simulink library "INP_SPR_ManOver"  (R2024b)
settings: Solver=VariableStepAuto  StartTime=0.0  StopTime=10.0  RelTol=1e-3
undefined symbols (not defined in the file): INP_SPR_p_SwtAccSprFrLeMan_na, INP_SPR_p_SwtAccSprFrRiMan_na, INP_SPR_p_SwtAccSprReLeMan_na, INP_SPR_p_SwtAccSprReRiMan_na, INP_SPR_s_AccSprFrLeMan_mps2, INP_SPR_s_AccSprFrRiMan_mps2, INP_SPR_s_AccSprLoLimFrLe_mps2, INP_SPR_s_AccSprLoLimFrRi_mps2, INP_SPR_s_AccSprLoLimReLe_mps2, INP_SPR_s_AccSprLoLimReRi_mps2, INP_SPR_s_AccSprReLeMan_mps2, INP_SPR_s_AccSprReRiMan_mps2, INP_SPR_s_AccSprUpLimFrLe_mps2, INP_SPR_s_AccSprUpLimFrRi_mps2, INP_SPR_s_AccSprUpLimReLe_mps2, INP_SPR_s_AccSprUpLimReRi_mps2
libraries: simulink x4
settings Model: Creator=blatak  LastModifiedBy=jmbsp

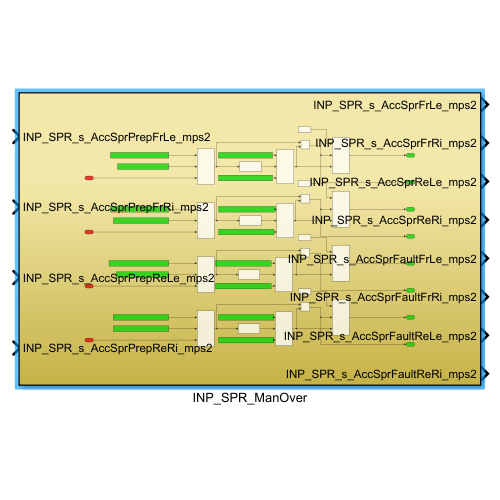
[thumbnail: Simulink's stored preview of the top-level diagram]
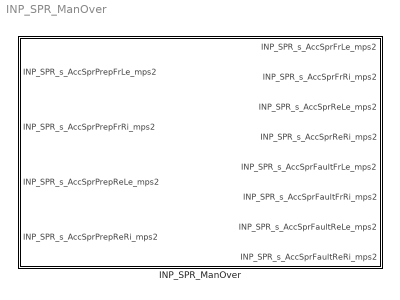
== system INP_SPR_ManOver ==
  INP_SPR_ManOver : Subsystem

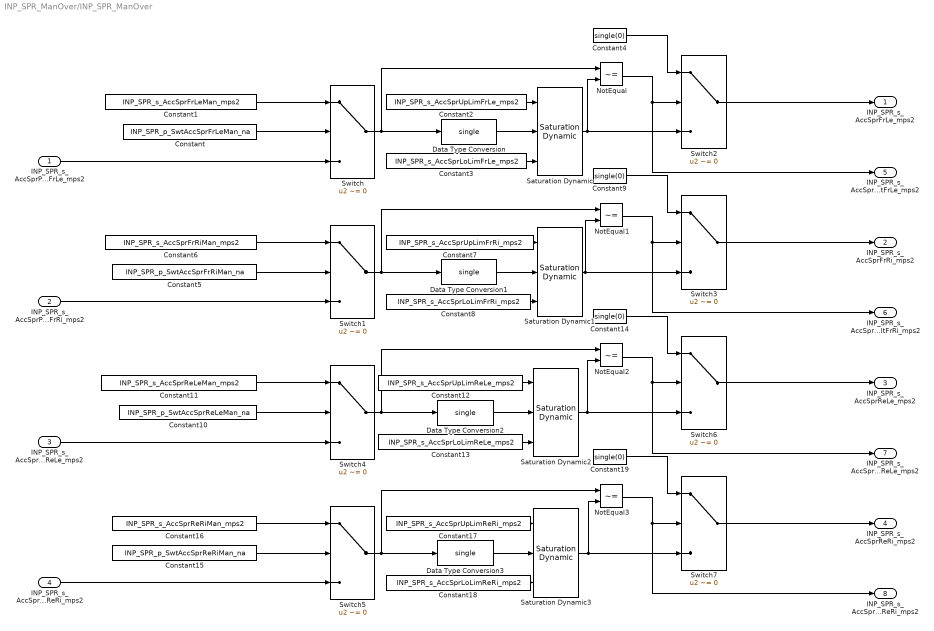
== system INP_SPR_ManOver/INP_SPR_ManOver ==
  INP_SPR_s_AccSprPrepFrLe_mps2 : Inport
  INP_SPR_s_AccSprPrepFrRi_mps2 : Inport  Port=2
  INP_SPR_s_AccSprPrepReLe_mps2 : Inport  Port=3
  INP_SPR_s_AccSprPrepReRi_mps2 : Inport  Port=4
  Constant : Constant  Description=|  Value=INP_SPR_p_SwtAccSprFrLeMan_na
      | Switch for manual override of the longitudinal acceleration value, if 1 instead the measured 
      | value the INP_IMU_p_ALgtVehMan_mps2 is used
  Constant1 : Constant  Description=|  Value=INP_SPR_s_AccSprFrLeMan_mps2
      | Value for longitudinal acceleration, which is used if the INP_IMU_p_SwtAXxxVehMan_na
      | is set to 1 instead of the measured value
  Constant10 : Constant  Description=|  Value=INP_SPR_p_SwtAccSprReLeMan_na
      | Switch for manual override of the longitudinal acceleration value, if 1 instead the measured 
      | value the INP_IMU_p_ALgtVehMan_mps2 is used
  Constant11 : Constant  Description=|  Value=INP_SPR_s_AccSprReLeMan_mps2
      | Value for longitudinal acceleration, which is used if the INP_IMU_p_SwtAXxxVehMan_na
      | is set to 1 instead of the measured value
  Constant12 : Constant  Description=Upper saturation limit for longitudinal acceleration  Value=INP_SPR_s_AccSprUpLimReLe_mps2
  Constant13 : Constant  Description=Lower saturation limit for longitudinal acceleration  Value=INP_SPR_s_AccSprLoLimReLe_mps2
  Constant{4,9,14,19} (4 alike) : Constant  Value=single(0)
  Constant15 : Constant  Description=|  Value=INP_SPR_p_SwtAccSprReRiMan_na
      | Switch for manual override of the longitudinal acceleration value, if 1 instead the measured 
      | value the INP_IMU_p_ALgtVehMan_mps2 is used
  Constant16 : Constant  Description=|  Value=INP_SPR_s_AccSprReRiMan_mps2
      | Value for longitudinal acceleration, which is used if the INP_IMU_p_SwtAXxxVehMan_na
      | is set to 1 instead of the measured value
  Constant17 : Constant  Description=Upper saturation limit for longitudinal acceleration  Value=INP_SPR_s_AccSprUpLimReRi_mps2
  Constant18 : Constant  Description=Lower saturation limit for longitudinal acceleration  Value=INP_SPR_s_AccSprLoLimReRi_mps2
  Constant2 : Constant  Description=Upper saturation limit for longitudinal acceleration  Value=INP_SPR_s_AccSprUpLimFrLe_mps2
  Constant3 : Constant  Description=Lower saturation limit for longitudinal acceleration  Value=INP_SPR_s_AccSprLoLimFrLe_mps2
  Constant5 : Constant  Description=|  Value=INP_SPR_p_SwtAccSprFrRiMan_na
      | Switch for manual override of the longitudinal acceleration value, if 1 instead the measured 
      | value the INP_IMU_p_ALgtVehMan_mps2 is used
  Constant6 : Constant  Description=|  Value=INP_SPR_s_AccSprFrRiMan_mps2
      | Value for longitudinal acceleration, which is used if the INP_IMU_p_SwtAXxxVehMan_na
      | is set to 1 instead of the measured value
  Constant7 : Constant  Description=Upper saturation limit for longitudinal acceleration  Value=INP_SPR_s_AccSprUpLimFrRi_mps2
  Constant8 : Constant  Description=Lower saturation limit for longitudinal acceleration  Value=INP_SPR_s_AccSprLoLimFrRi_mps2
  Data Type Conversion{,1..3} (4 alike) : DataTypeConversion  OutDataTypeStr=single  SaturateOnIntegerOverflow=off  RndMeth=Floor
  NotEqual{,1..3} (4 alike) : RelationalOperator  Operator=~=  OutDataTypeStr=boolean  RndMeth=Simplest  InputSameDT=off
  Saturation Dynamic{,1..3} (4 alike) : simulink/Discontinuities/Saturation Dynamic  OutMin=[]  OutMax=[]  OutDataTypeStr=Inherit: Same as second input  OutDataType=fixdt(1, 16)  OutScaling=2^-10  DoSatur=off
  Switch{,1..7} (8 alike) : Switch  Criteria=u2 ~= 0  SaturateOnIntegerOverflow=off  InputSameDT=off
  INP_SPR_s_AccSprFrLe_mps2 : Outport
  INP_SPR_s_AccSprFrRi_mps2 : Outport  Port=2
  INP_SPR_s_AccSprReLe_mps2 : Outport  Port=3
  INP_SPR_s_AccSprReRi_mps2 : Outport  Port=4
  INP_SPR_s_AccSprFaultFrLe_mps2 : Outport  Port=5
  INP_SPR_s_AccSprFaultFrRi_mps2 : Outport  Port=6
  INP_SPR_s_AccSprFaultReLe_mps2 : Outport  Port=7
  INP_SPR_s_AccSprFaultReRi_mps2 : Outport  Port=8
  wires:
  Constant7/1 -> Saturation Dynamic1/1
  NotEqual1/1 -> INP_SPR_s_AccSprFaultFrRi_mps2/1, Switch3/2
  Saturation Dynamic2/1 -> Switch6/3, NotEqual2/2
  Constant6/1 -> Switch1/1
  Data Type Conversion/1 -> Saturation Dynamic/2
  NotEqual/1 -> INP_SPR_s_AccSprFaultFrLe_mps2/1, Switch2/2
  INP_SPR_s_AccSprPrepReRi_mps2/1 -> Switch5/3
  Saturation Dynamic1/1 -> Switch3/3, NotEqual1/2
  Constant1/1 -> Switch/1
  NotEqual2/1 -> INP_SPR_s_AccSprFaultReLe_mps2/1, Switch6/2
  Constant13/1 -> Saturation Dynamic2/3
  Constant16/1 -> Switch5/1
  INP_SPR_s_AccSprPrepFrRi_mps2/1 -> Switch1/3
  Constant17/1 -> Saturation Dynamic3/1
  Switch4/1 -> NotEqual2/1, Data Type Conversion2/1
  Data Type Conversion2/1 -> Saturation Dynamic2/2
  Saturation Dynamic3/1 -> Switch7/3, NotEqual3/2
  Constant14/1 -> Switch6/1
  Constant10/1 -> Switch4/2
  Switch2/1 -> INP_SPR_s_AccSprFrLe_mps2/1
  Constant3/1 -> Saturation Dynamic/3
  Constant12/1 -> Saturation Dynamic2/1
  INP_SPR_s_AccSprPrepReLe_mps2/1 -> Switch4/3
  Saturation Dynamic/1 -> Switch2/3, NotEqual/2
  Switch6/1 -> INP_SPR_s_AccSprReLe_mps2/1
  Constant8/1 -> Saturation Dynamic1/3
  Switch1/1 -> NotEqual1/1, Data Type Conversion1/1
  Switch/1 -> NotEqual/1, Data Type Conversion/1
  Constant/1 -> Switch/2
  NotEqual3/1 -> INP_SPR_s_AccSprFaultReRi_mps2/1, Switch7/2
  Constant18/1 -> Saturation Dynamic3/3
  Constant2/1 -> Saturation Dynamic/1
  Switch5/1 -> NotEqual3/1, Data Type Conversion3/1
  Constant11/1 -> Switch4/1
  Data Type Conversion1/1 -> Saturation Dynamic1/2
  Data Type Conversion3/1 -> Saturation Dynamic3/2
  INP_SPR_s_AccSprPrepFrLe_mps2/1 -> Switch/3
  Constant15/1 -> Switch5/2
  Switch7/1 -> INP_SPR_s_AccSprReRi_mps2/1
  Switch3/1 -> INP_SPR_s_AccSprFrRi_mps2/1
  Constant5/1 -> Switch1/2
  Constant9/1 -> Switch3/1
  Constant19/1 -> Switch7/1
  Constant4/1 -> Switch2/1
